simulink library "RxTxFixedPointLibrary"  (R2018a)
settings: Solver=VariableStepAuto  StartTime=0.0  StopTime=10.0  RelTol=1e-3
values from neighbouring files (symbols this model uses):
  AGCBarkerSymbols = 160 + 28    (= 188)    [modelSettings.m]
  coeff = rcosdesign(beta, span, sps, 'sqrt') * filterGain    [modelSettings.m]
  crcDecodeLag = length(crc32Poly) - 1 + 2    [modelSettings.m]
  CRCGeneratorLag = 34    [modelSettings.m]
  EQTrainingSymbols = 250    [modelSettings.m]
  K1 = fi(K1, 0)    [modelSettings.m]
  K2 = fi(K2, 0)    [modelSettings.m]
  numHeaderBits = 16    [modelSettings.m]
  numTrainingSamples = 250    [modelSettings.m]
  pLen = uint16(length(PreambleBarkersBits))    [modelSettings.m]
  RadioSampleRate = 1e6    (= 1000000)    [modelSettings.m]
  samplesPerSymbol = 4    [modelSettings.m]
  VibertiTracebackLength = 34 + 0    (= 34)    [modelSettings.m]
  xPreambleSeq = hPSKModTrain(seq)    [modelSettings.m]
undefined symbols (not defined in the file or in its folder): j
libraries: simulink x25, dsphdlfiltering x20, hdlsllib x10, commseqgen3 x4, commdigbbndpm3 x3, commcrc2 x2, commcnvcod2 x2, dspstat3 x1, commfilt2 x1, dspsigops x1
(part 2 of 3)

== system RxTxFixedPointLibrary/Receiver_HDL/Frame Recover/Barker Locate/Measure Phase Ambiguity ==
  data : Inport  OutDataTypeStr=int16
  trigger : Inport  Port=2
  validIn : Inport  Port=3
  Find Max and Set Output Shift : Subsystem
  HDL Opt Complex FIR4 : Subsystem  mask{Taps=xPreambleSeq(end:-1:1).'}
  HDL Opt Complex FIR5 : Subsystem  mask{Taps=exp(-j*pi/2).*xPreambleSeq(end:-1:1).'}
  HDL Opt Complex FIR6 : Subsystem  mask{Taps=exp(-j*pi).*xPreambleSeq(end:-1:1).'}
  HDL Opt Complex FIR7 : Subsystem  mask{Taps=exp(-j*pi*3/2).*xPreambleSeq(end:-1:1).'}
  Logical Operator : Logic  Inputs=5  AllPortsSameDT=off  OutDataTypeStr=boolean
  PA : Outport  InitialOutput=0
  wires:
  trigger/1 -> Logical Operator/5
  Logical Operator/1 -> Find Max and Set Output Shift/Enable
  HDL Opt Complex FIR7/2(validOut) -> Logical Operator/4
  HDL Opt Complex FIR6/2(validOut) -> Logical Operator/3
  HDL Opt Complex FIR5/2(validOut) -> Logical Operator/2
  HDL Opt Complex FIR4/2(validOut) -> Logical Operator/1
  validIn/1 -> HDL Opt Complex FIR6/2(validIn), HDL Opt Complex FIR7/2(validIn), HDL Opt Complex FIR5/2(validIn), HDL Opt Complex FIR4/2(validIn)
  Find Max and Set Output Shift/1(Out1) -> PA/1
  HDL Opt Complex FIR7/1(Out1) -> Find Max and Set Output Shift/4(In5)
  HDL Opt Complex FIR6/1(Out1) -> Find Max and Set Output Shift/3(In4)
  HDL Opt Complex FIR5/1(Out1) -> Find Max and Set Output Shift/2(In2)
  HDL Opt Complex FIR4/1(Out1) -> Find Max and Set Output Shift/1(In1)
  data/1 -> HDL Opt Complex FIR6/1(In1), HDL Opt Complex FIR7/1(In1), HDL Opt Complex FIR5/1(In1), HDL Opt Complex FIR4/1(In1)

== system RxTxFixedPointLibrary/Receiver_HDL/Frame Recover/Equalization and Demodulation/2 Bit Descrambler ==
  note: This is a special Descrambler which can process 2 bits at a time
  u1 : Inport
  reset : Inport  Port=2
  Demux1 : Demux  Outputs=2
  MATLAB Function : MATLAB Function  TreatAsAtomicUnit=on
  Mux : Mux  Inputs=2
  Selector1 : Selector  IndexOptions=Index vector (dialog)  Indices=find(polynom(2:end))  OutputSizes=1
  Selector2 : Selector  IndexOptions=Index vector (dialog)  Indices=find(polynom(2:end))  OutputSizes=1
  input_xor1 : Logic  Operator=XOR  IconShape=distinctive  AllPortsSameDT=off  OutDataTypeStr=boolean
  input_xor2 : Logic  Operator=XOR  IconShape=distinctive  AllPortsSameDT=off  OutDataTypeStr=boolean
  state_xor1 : Logic  Operator=XOR  Inputs=1  IconShape=distinctive  AllPortsSameDT=off  OutDataTypeStr=boolean
  state_xor2 : Logic  Operator=XOR  Inputs=1  IconShape=distinctive  AllPortsSameDT=off  OutDataTypeStr=boolean
  y1 : Outport  InitialOutput=0
  wires:
  Demux1/2 -> input_xor2/2  "data_in"
  Demux1/1 -> input_xor1/2
  Selector2/1 -> state_xor2/1
  Selector1/1 -> state_xor1/1
  input_xor1/1 -> Mux/1
  input_xor2/1 -> Mux/2
  state_xor2/1 -> input_xor2/1
  state_xor1/1 -> input_xor1/1
  Mux/1 -> y1/1
  MATLAB Function/2(bufferB) -> Selector2/1
  MATLAB Function/1(bufferA) -> Selector1/1
  reset/1 -> MATLAB Function/2(reset)
  u1/1 -> MATLAB Function/1(bits), Demux1/1

== system RxTxFixedPointLibrary/Receiver_HDL/Frame Recover/Equalization and Demodulation/DFE ==
  note: Generate training sequence when barker is found
  note: refTap=0 to disableEQ
  Trigger : Inport  PortDimensions=1
  data : Inport  Port=2  PortDimensions=1
      settings: SignalType=complex
  EQmu : Inport  Port=3
  DFE : Subsystem  mask{numFTaps=5, numBTaps=3, mu=0.01, refTap=2}
      mask prompts: numFTaps "Num Forward Taps"; numBTaps "Num Backward Taps"; mu "Step Size"; refTap "Reference Tap"
  Delay data so DFE can reset : Delay  DelayLength=1
  Delay ref so DFE can reset : Delay  DelayLength=1
  Equalizer : MATLAB Function  Commented=on  TreatAsAtomicUnit=on
  PN Sequence Generator : commseqgen3/PN Sequence Generator  poly='z^5 + z^3 + z^1 + 1'  ini_sta=[1 1 1 0 0]  outBitMaskSource=Dialog parameter  shift=0  outVarSiz=off  maxOutSizeMode=Dialog parameter  maxOutSize=[10 1]  Ts=-1  sampPerFrame=1  reset=on  bitPackedOutputs=on  outDataType=Smallest unsigned integer  numPackedBits=2  bitPackDataSigned=off  bitPackedOutDType=Smallest integer
      settings: SourceProductName=Communications System Toolbox
  Packeted To Unpacked : Subsystem
  QPSK Modulator Baseband : commdigbbndpm3/QPSK Modulator Baseband  InType=Bit  Enc=Binary  Ph=pi/4  outDtype=Fixed-point  outWordLen=16  outUDDataType=sfix(16)  outFracLenMode=User-defined  outFracLen=15  outDataTypeStr=fixdt(1,16,15)  outLastDataTypeStr=fixdt(1,16,15)
  Terminator1 : Terminator
  dataEQed : Outport
  start : Outport  Port=2
  wires:
  EQmu/1 -> DFE/4(EQmu)
  Delay ref so DFE can reset/1 -> DFE/3(training)
  Delay data so DFE can reset/1 -> DFE/2(dataIn)
  DFE/1(eqOut) -> dataEQed/1
  DFE/2(err) -> Terminator1/1
  Trigger/1 -> PN Sequence Generator/1, DFE/1(reset)
  DFE/3(start) -> start/1
  QPSK Modulator Baseband/1 -> Delay ref so DFE can reset/1
  Packeted To Unpacked/1(Out1) -> QPSK Modulator Baseband/1
  PN Sequence Generator/1 -> Packeted To Unpacked/1(In1)
  data/1 -> Delay data so DFE can reset/1

== system RxTxFixedPointLibrary/Receiver_HDL/Frame Recover/Frequency Recovery/Lock Detector ==
  ped : Inport
  Compare To Constant : simulink/Logic and Bit Operations/Compare To Constant  relop=<=  const=Threshold*WindowLength  OutDataTypeStr=boolean
  MATLAB Function : MATLAB Function  TreatAsAtomicUnit=on
  PED Error : Scope  Commented=on  NumInputPorts=3
  Pipeline Delay : Delay  DelayLength=1
  Sum of Elements : Sum  Inputs=+
  Tapped Delay : simulink/Discrete/Tapped Delay  vinit=0.0  samptime=-1  NumDelays=WindowLength  DelayOrder=Oldest  includeCurrent=off
  lock : Outport
  wires:
  ped/1 -> Pipeline Delay/1
  Tapped Delay/1 -> Sum of Elements/1
  Sum of Elements/1 -> PED Error/3, Compare To Constant/1
  Compare To Constant/1 -> lock/1, PED Error/2
  MATLAB Function/1(y) -> PED Error/1, Tapped Delay/1
  Pipeline Delay/1 -> MATLAB Function/1(u)

== system RxTxFixedPointLibrary/Receiver_HDL/Frame Recover/Frequency Recovery/Loop Filter ==
  note: Proportional-plus-Integrator Loop Filter,
      | Infinite DC Response to guarantee convergence
  note: This inflation is necessary
  e : Inport
  Add1 : Sum  RndMeth=Nearest  OutDataTypeStr=Inherit: Same as first input
  Add2 : Sum  OutDataTypeStr=Inherit: Same as first input
  Data Type Conversion : DataTypeConversion  OutDataTypeStr=fixdt(1,25,20)
  Delay : Delay  DelayLength=1
  Delay3 : Delay  DelayLength=1
  Delay4 : Delay  DelayLength=1
  K1 : Gain  Gain=K2  OutDataTypeStr=Inherit: Same as input
  K2 : Gain  Gain=K1  OutDataTypeStr=Inherit: Same as input
  Sum2 : Sum  OutDataTypeStr=Inherit: Same as first input
  v : Outport
  wires:
  Data Type Conversion/1 -> v/1
  Add2/1 -> Data Type Conversion/1, Delay4/1
  Delay4/1 -> Add2/2
  Delay3/1 -> Add2/1
  Sum2/1 -> Delay3/1
  Delay/1 -> Add1/1
  K2/1 -> Add1/2, Delay/1
  e/1 -> K1/1, K2/1
  Add1/1 -> Sum2/2
  K1/1 -> Sum2/1

== system RxTxFixedPointLibrary/Receiver_HDL/Frame Recover/Frequency Recovery/Loop Filter Configurable ==
  note: Proportional-plus-Integrator Loop Filter,
      | Infinite DC Response to guarantee convergence
  note: This inflation is necessary
  e : Inport
  LoopBW : Inport  Port=2
  Add1 : Sum  RndMeth=Nearest  OutDataTypeStr=Inherit: Same as first input
  Add2 : Sum  OutDataTypeStr=Inherit: Same as first input
  Data Type Conversion : DataTypeConversion  OutDataTypeStr=fixdt(1,25,20)
  Delay : Delay  DelayLength=1
  Delay3 : Delay  DelayLength=1
  Delay4 : Delay  DelayLength=1
  Direct Lookup Table (n-D) : LookupNDDirect  NumberOfTableDimensions=1  Table=K1  DiagnosticForOutOfRangeInput=Error
  Direct Lookup Table (n-D)1 : LookupNDDirect  NumberOfTableDimensions=1  Table=K2  DiagnosticForOutOfRangeInput=Error
  Product : Product  OutDataTypeStr=Inherit: Same as first input
  Product1 : Product  OutDataTypeStr=Inherit: Same as first input
  Sum2 : Sum  OutDataTypeStr=Inherit: Same as first input
  v : Outport
  wires:
  LoopBW/1 -> Direct Lookup Table (n-D)1/1, Direct Lookup Table (n-D)/1
  Direct Lookup Table (n-D)1/1 -> Product1/2
  Direct Lookup Table (n-D)/1 -> Product/2
  Data Type Conversion/1 -> v/1
  Add2/1 -> Data Type Conversion/1, Delay4/1
  Delay4/1 -> Add2/2
  Delay3/1 -> Add2/1
  Sum2/1 -> Delay3/1
  Delay/1 -> Add1/1
  Product1/1 -> Add1/2, Delay/1
  e/1 -> Product/1, Product1/1
  Add1/1 -> Sum2/2
  Product/1 -> Sum2/1

== system RxTxFixedPointLibrary/Receiver_HDL/Frame Recover/Frequency Recovery/Phase Shift FP ==
  note: Sign Comes from original
      | loop filter design
  In1 : Inport
  Phi : Inport  Port=2
  Cosine HDL Optimized : hdlsllib/Lookup Tables/Cosine HDL Optimized  OutputFormula=exp(j*2*pi*u)  NumDataPoints=256  TableDataTypeStr=fixdt(0,31,20)  SimulateLUTROMDelay=off
      settings: SourceProductName=HDL Coder  SourceProductBaseCode=HD
  Gain : Gain  Gain=-1/(2*pi)  ParamDataTypeStr=fixdt(1,25,20)  OutDataTypeStr=fixdt(1,16,12)  SaturateOnIntegerOverflow=on
  Product : Product  OutDataTypeStr=fixdt(1,16,13)  SaturateOnIntegerOverflow=on
  Out1 : Outport
  wires:
  Gain/1 -> Cosine HDL Optimized/1
  Phi/1 -> Gain/1
  In1/1 -> Product/1
  Cosine HDL Optimized/1 -> Product/2
  Product/1 -> Out1/1

== system RxTxFixedPointLibrary/Receiver_HDL/Frame Recover/Gardner Timing Recovery/Gardner TED Blocks ==
  note: This is for QPSK and 4 SamplesPerSymbol ONLY
  note: An input of 4 should not
      | happen unless the input is all zeros
  data : Inport
  strobe : Inport  Port=2
  Add : Sum  OutDataTypeStr=fixdt(1,16,15)
  Check Only Strobe Condition : simulink/Logic and Bit Operations/Compare To Constant  relop===  const=uint8(1)  OutDataTypeStr=boolean
  Complex to Real-Imag : ComplexToRealImag
  Constant : Constant  Value=0  OutDataTypeStr=Inherit: Inherit via back propagation  SampleTime=-1
  Display : Display
  Imag Error : Subsystem
  Logical Operator : Logic  AllPortsSameDT=off  OutDataTypeStr=boolean
  Map [0,1,2,3,4] to [0,1,2,2,2] : LookupNDDirect  NumberOfTableDimensions=1  Table=[0 1 2 2 2]  DiagnosticForOutOfRangeInput=Error  TableDataTypeStr=uint8
  Real Error : Subsystem
  Strobe Buffer1 : simulink/Discrete/Tapped Delay  vinit=0.0  samptime=-1  NumDelays=samplesPerSymbol-1  DelayOrder=Oldest  includeCurrent=on
  Sum of Elements1 : Sum  Inputs=+  OutDataTypeStr=int8
  Switch : Switch  Criteria=u2 ~= 0  SaturateOnIntegerOverflow=on
  e : Outport
  wires:
  Logical Operator/1 -> Switch/2
  Add/1 -> Switch/1
  Imag Error/1(Out1) -> Add/2
  Real Error/1(Out1) -> Add/1
  Strobe Buffer1/1 -> Sum of Elements1/1
  Map [0,1,2,3,4] to [0,1,2,2,2]/1 -> Real Error/2(strobe sum), Imag Error/2(strobe sum)
  data/1 -> Complex to Real-Imag/1
  Complex to Real-Imag/1 -> Real Error/1(data)
  Constant/1 -> Switch/3
  Check Only Strobe Condition/1 -> Logical Operator/1
  Sum of Elements1/1 -> Map [0,1,2,3,4] to [0,1,2,2,2]/1, Check Only Strobe Condition/1, Display/1
  Complex to Real-Imag/2 -> Imag Error/1(data)
  strobe/1 -> Logical Operator/2, Strobe Buffer1/1
  Switch/1 -> e/1

== system RxTxFixedPointLibrary/Receiver_HDL/Frame Recover/Gardner Timing Recovery/InterpControl_Blocks1 ==
  note: Mu is always positive
  note: e<<1/SPS
  e : Inport
  1/SPS1 : Constant  Value=fi(1/samplesPerSymbol,0,2,2)  OutDataTypeStr=fixdt(0,2,2)  SampleTime=-1
  Add1 : Sum  OutDataTypeStr=fixdt(0,16,16)
  Calculate New mu : Subsystem
  Display{,1..3} (4 alike) : Display
  Mod 1 : Subsystem
  NCOCounter State : Delay  DelayLength=1  InitialCondition=0
  Subtract1 : Sum  Inputs=-+  OutDataTypeStr=Inherit: Same as first input
  Update mu on strobe : Switch  Criteria=u2 > Threshold
  saved mu : Delay  DelayLength=1
  strobe == W>NCOCounter : RelationalOperator  Operator=>  OutDataTypeStr=boolean  RndMeth=Nearest
  strobe : Outport
  mu : Outport  Port=2
  wires:
  Add1/1 -> Subtract1/1, Display2/1, strobe == W>NCOCounter/1, Calculate New mu/1(W)
  1/SPS1/1 -> Add1/2
  Mod 1/1(Out1) -> NCOCounter State/1
  Subtract1/1 -> Mod 1/1(In1)
  NCOCounter State/1 -> Calculate New mu/2(NCOCounter), strobe == W>NCOCounter/2, Display1/1, Subtract1/2
  e/1 -> Add1/1
  Calculate New mu/1(mu) -> Update mu on strobe/1, Display/1
  saved mu/1 -> Update mu on strobe/3
  Update mu on strobe/1 -> saved mu/1, mu/1, Display3/1
  strobe == W>NCOCounter/1 -> strobe/1, Update mu on strobe/2

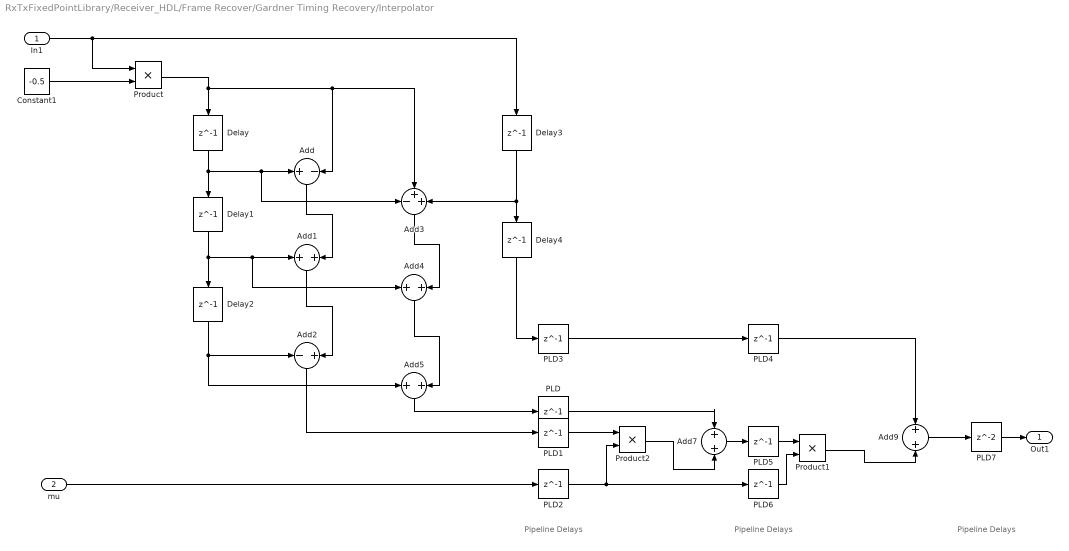
== system RxTxFixedPointLibrary/Receiver_HDL/Frame Recover/Gardner Timing Recovery/Interpolator ==
  note: Pipeline Delays
  note: Pipeline Delays
  note: Pipeline Delays
  In1 : Inport
  mu : Inport  Port=2
  Add : Sum  Inputs=+-  OutDataTypeStr=Inherit: Same as first input
  Add{1,4..5,7} (4 alike) : Sum
  Add2 : Sum  Inputs=-+
  Add3 : Sum  Inputs=-++
  Add9 : Sum  OutDataTypeStr=fixdt(1,16,10)
  Constant1 : Constant  Value=-0.5  OutDataTypeStr=fixdt(1,2,2)  SampleTime=-1
  Delay{,1..4} (5 alike) : Delay  DelayLength=1
  PLD{,1..6} (7 alike) : Delay  DelayLength=1
  PLD7 : Delay
  Product : Product  OutDataTypeStr=fixdt(1,16,14)
  Product1 : Product
  Product2 : Product  OutDataTypeStr=fixdt(1,16,10)
  Out1 : Outport
  wires:
  PLD7/1 -> Out1/1
  PLD6/1 -> Product1/2
  PLD5/1 -> Product1/1
  PLD4/1 -> Add9/1
  PLD3/1 -> PLD4/1
  PLD2/1 -> PLD6/1, Product2/2
  PLD1/1 -> Product2/1
  PLD/1 -> Add7/1
  Constant1/1 -> Product/2
  Product1/1 -> Add9/2
  Add7/1 -> PLD5/1
  Delay4/1 -> PLD3/1
  Delay3/1 -> Add3/3, Delay4/1
  Add9/1 -> PLD7/1
  Product2/1 -> Add7/2
  Add5/1 -> PLD/1
  mu/1 -> PLD2/1
  Add2/1 -> PLD1/1
  Add4/1 -> Add5/2
  Add3/1 -> Add4/2
  Add1/1 -> Add2/2
  Delay2/1 -> Add2/1, Add5/1
  Add/1 -> Add1/2
  Delay1/1 -> Delay2/1, Add1/1, Add4/1
  Delay/1 -> Delay1/1, Add/1, Add3/1
  Product/1 -> Delay/1, Add/2, Add3/2
  In1/1 -> Product/1, Delay3/1

== system RxTxFixedPointLibrary/Receiver_HDL/Frame Recover/Gardner Timing Recovery/LoopFilter1 ==
  e : Inport
  Delay1 : Delay  DelayLength=1
  Delay2 : Delay  DelayLength=1
  Proportional Gain : Gain  Gain=fi(ProportionalGain,1,16,15)  OutDataTypeStr=fixdt(1,16,24)
  v : Outport
  wires:
  Delay1/1 -> v/1
  Delay2/1 -> Proportional Gain/1
  Proportional Gain/1 -> Delay1/1
  e/1 -> Delay2/1

== system RxTxFixedPointLibrary/Receiver_HDL/Frame Recover/Gardner Timing Recovery/TED Lock Detector ==
  ted : Inport
  Compare To Constant : simulink/Logic and Bit Operations/Compare To Constant  relop=<=  const=Threshold*WindowLength  OutDataTypeStr=boolean
  MATLAB Function : MATLAB Function  TreatAsAtomicUnit=on
  Pipeline Delay : Delay  DelayLength=1
  Sum of Elements : Sum  Inputs=+
  TED Error : Scope  Commented=on  NumInputPorts=3
  Tapped Delay : simulink/Discrete/Tapped Delay  vinit=0.0  samptime=-1  NumDelays=WindowLength  DelayOrder=Oldest  includeCurrent=off
  lock : Outport
  wires:
  ted/1 -> Pipeline Delay/1
  Tapped Delay/1 -> Sum of Elements/1
  Sum of Elements/1 -> TED Error/3, Compare To Constant/1
  Compare To Constant/1 -> lock/1, TED Error/2
  MATLAB Function/1(y) -> TED Error/1, Tapped Delay/1
  Pipeline Delay/1 -> MATLAB Function/1(u)

== system RxTxFixedPointLibrary/Receiver_HDL/Frame Recover/Manage Error Signals/Subsystem ==
  <status> : Inport
  <s1> : Inport  Port=2
  <s2> : Inport  Port=3
  Enable : EnablePort
  DEBUG: Header : MATLAB Function  Commented=on  TreatAsAtomicUnit=on
  wires:
  <s1>/1 -> DEBUG: Header/2(h1)
  <status>/1 -> DEBUG: Header/1(status)
  <s2>/1 -> DEBUG: Header/3(h2)

== system RxTxFixedPointLibrary/Receiver_HDL/Viterbi Decode/Buffer/DEBUG: Vitberi Check ==
  In1 : Inport
  In2 : Inport  Port=2
  In3 : Inport  Port=3
  In4 : Inport  Port=4
  Allow Viterbi Reset2 : Delay  DelayLength=1
  Allow Viterbi Reset3 : Delay  DelayLength=34
  Allow Viterbi Reset4 : Delay  DelayLength=1
  MATLAB Function2 : MATLAB Function  TreatAsAtomicUnit=on
  wires:
  In3/1 -> Allow Viterbi Reset2/1
  In1/1 -> MATLAB Function2/1(bits)
  In2/1 -> Allow Viterbi Reset4/1
  Allow Viterbi Reset2/1 -> MATLAB Function2/3(reset)
  In4/1 -> Allow Viterbi Reset3/1
  Allow Viterbi Reset3/1 -> MATLAB Function2/4(crc)
  Allow Viterbi Reset4/1 -> MATLAB Function2/2(enable)

== system RxTxFixedPointLibrary/Transmitter_HDL/Packet Generation/Payload/Enable Latch ==
  note: This block will latch when start flag is high and then latch low when end flag arrives
  mode : Inport
  start : Inport  Port=2
  end : Inport  Port=3
  Compare To Constant : simulink/Logic and Bit Operations/Compare To Constant  relop=>=  const=uint8(1)  OutDataTypeStr=boolean
  Compare To Constant1 : simulink/Logic and Bit Operations/Compare To Constant  relop===  const=uint8(1)  OutDataTypeStr=boolean
  HDL Counter1 : hdlsllib/Sources/HDL Counter  CountType=Count limited  CountInit=0  CountStep=1  CountMax=1  CountFromType=Initial value  CountFrom=0  CountResetPort=on  CountLoadPort=off  CountEnbPort=on  CountDirPort=off  CountDataType=Unsigned  CountWordLen=8  CountFracLen=0  CountSampTime=1
      settings: SourceProductBaseCode=HD
  Logical Operator : Logic  AllPortsSameDT=off  OutDataTypeStr=boolean
  Logical Operator1 : Logic  AllPortsSameDT=off  OutDataTypeStr=boolean
  Logical Operator2 : Logic  Operator=OR  AllPortsSameDT=off  OutDataTypeStr=boolean
  MATLAB Function : MATLAB Function  Commented=on  TreatAsAtomicUnit=on
  Terminator : Terminator  Commented=on
  valid : Outport
  wires:
  mode/1 -> Compare To Constant/1
  Compare To Constant/1 -> Logical Operator1/1, Logical Operator/1
  start/1 -> MATLAB Function/1(startpacket), Logical Operator/2
  end/1 -> MATLAB Function/2(endpacket), Logical Operator1/2
  HDL Counter1/1 -> Compare To Constant1/1
  Logical Operator1/1 -> HDL Counter1/1
  Logical Operator/1 -> Logical Operator2/1, HDL Counter1/2
  Compare To Constant1/1 -> Logical Operator2/2
  MATLAB Function/1(outEnable) -> Terminator/1
  Logical Operator2/1 -> valid/1

== system RxTxFixedPointLibrary/Transmitter_HDL/Packet Generation/Payload/HDL Scrambler 2 bits ==
  bitsIn : Inport
  reset : Inport  Port=2
  Buffer Manage : MATLAB Function  TreatAsAtomicUnit=on
  Delay : Delay  DelayLength=1  InitialCondition=false
  Delay1 : Delay  DelayLength=1  InitialCondition=false
  Demux : Demux  Outputs=2
  Display1 : Display
  Display3 : Display
  Mux : Mux  Inputs=2
  Mux1 : Mux  Inputs=2
  Selector : Selector  IndexOptions=Index vector (dialog)  Indices=find(poly(2:end))  OutputSizes=1
  Selector1 : Selector  IndexOptions=Index vector (dialog)  Indices=1+find(poly(2:end))  OutputSizes=1
  state_xor1 : Logic  Operator=XOR  IconShape=distinctive  AllPortsSameDT=off  OutDataTypeStr=boolean
  state_xor2 : Logic  Operator=XOR  Inputs=1  IconShape=distinctive  AllPortsSameDT=off  OutDataTypeStr=boolean
  state_xor3 : Logic  Operator=XOR  Inputs=1  IconShape=distinctive  AllPortsSameDT=off  OutDataTypeStr=boolean
  state_xor4 : Logic  Operator=XOR  IconShape=distinctive  AllPortsSameDT=off  OutDataTypeStr=boolean
  bitsOut : Outport
  wires:
  bitsIn/1 -> Display1/1, Demux/1
  Selector/1 -> state_xor2/1
  state_xor2/1 -> Display3/1, state_xor1/1
  Demux/1 -> state_xor1/2
  state_xor1/1 -> Mux1/2, Mux/1, Delay/1
  Mux/1 -> bitsOut/1
  Mux1/1 -> Selector1/1
  Buffer Manage/1(outBuffer) -> Mux1/1, Selector/1
  Selector1/1 -> state_xor3/1
  state_xor3/1 -> state_xor4/1
  Demux/2 -> state_xor4/2
  state_xor4/1 -> Delay1/1, Mux/2
  Delay/1 -> Buffer Manage/1(bit1)
  reset/1 -> Buffer Manage/3(reset)
  Delay1/1 -> Buffer Manage/2(bit2)

== system RxTxFixedPointLibrary/Transmitter_HDL/Packet Generation/Payload/Subsystem ==
  In1 : Inport
  In2 : Inport  Port=2
  Logical Operator : Logic  Operator=OR  Inputs=3  AllPortsSameDT=off  OutDataTypeStr=boolean
  MATLAB Function3 : MATLAB Function  TreatAsAtomicUnit=on
  Out1 : Outport
  wires:
  In2/1 -> Logical Operator/3, MATLAB Function3/2(done)
  In1/1 -> Logical Operator/1, MATLAB Function3/1(start)
  MATLAB Function3/1(enable) -> Logical Operator/2
  Logical Operator/1 -> Out1/1

== system RxTxFixedPointLibrary/Transmitter_HDL/Packet Generation/Preamble/Unpack1 ==
  In1 : Inport
  Data Type Conversion : DataTypeConversion  OutDataTypeStr=boolean
  Extract Bits : simulink/Logic and Bit Operations/Extract Bits  bitsToExtract=Range of bits  numBits=8  bitIdxRange=[1]  outScalingMode=Treat bit field as an integer
      settings: SourceProductName=Simulink
  Extract Bits1 : simulink/Logic and Bit Operations/Extract Bits  bitsToExtract=Range of bits  numBits=8  bitIdxRange=[0]  outScalingMode=Treat bit field as an integer
      settings: SourceProductName=Simulink
  Vector Concatenate : Concatenate
  Out1 : Outport
  wires:
  In1/1 -> Extract Bits1/1, Extract Bits/1
  Extract Bits/1 -> Vector Concatenate/1
  Extract Bits1/1 -> Vector Concatenate/2
  Vector Concatenate/1 -> Data Type Conversion/1
  Data Type Conversion/1 -> Out1/1

== system RxTxFixedPointLibrary/Transmitter_HDL/Packet Generation/Random Data/Unpack ==
  In1 : Inport
  Data Type Conversion : DataTypeConversion  OutDataTypeStr=boolean
  Extract Bits : simulink/Logic and Bit Operations/Extract Bits  bitsToExtract=Range of bits  numBits=8  bitIdxRange=[0]  outScalingMode=Treat bit field as an integer
      settings: SourceProductName=Simulink
  Extract Bits1 : simulink/Logic and Bit Operations/Extract Bits  bitsToExtract=Range of bits  numBits=8  bitIdxRange=[1]  outScalingMode=Treat bit field as an integer
      settings: SourceProductName=Simulink
  Vector Concatenate : Concatenate
  Out1 : Outport
  wires:
  In1/1 -> Extract Bits1/1, Extract Bits/1
  Extract Bits/1 -> Vector Concatenate/1
  Extract Bits1/1 -> Vector Concatenate/2
  Vector Concatenate/1 -> Data Type Conversion/1
  Data Type Conversion/1 -> Out1/1

== system RxTxFixedPointLibrary/Receiver_HDL/Frame Recover/Barker Locate/Measure Phase Ambiguity/Find Max and Set Output Shift ==
  In1 : Inport
  In2 : Inport  Port=2
  In4 : Inport  Port=3
  In5 : Inport  Port=4
  Enable : EnablePort
  Complex to Real-Imag{,1..3} (4 alike) : ComplexToRealImag  Output=Imag
  Direct Lookup Table (n-D) : LookupNDDirect  NumberOfTableDimensions=1  Table=exp(-(0:pi/2:(pi*3/2)) .* 1i).'  DiagnosticForOutOfRangeInput=Error  TableDataTypeStr=fixdt(1,16,13)
  Display : Display
  Display1 : Display
  Maximum : dspstat3/Maximum  operation=maximum  fcn=Index  indexBase=Zero  operateOver=Each column  Dimension=1  InputProcessing=Columns as channels (frame based)  reset=None  roiEnable=off  roiType=Rectangles  roiPortion=Entire ROI  roiOutput=Individual statistics for each ROI  roiFlag=off  roundingMode=Floor  overflowMode=off  accumDataTypeStr=Inherit: Same as product output  accumLastDataTypeStr=Inherit: Same as product output
  Vector Concatenate : Concatenate  NumInputs=4
  Vector Concatenate1 : Concatenate  NumInputs=4
  Out1 : Outport  InitialOutput=0
  wires:
  Complex to Real-Imag/1 -> Vector Concatenate/1
  Complex to Real-Imag2/1 -> Vector Concatenate/3
  Complex to Real-Imag3/1 -> Vector Concatenate/4
  Complex to Real-Imag1/1 -> Vector Concatenate/2
  Vector Concatenate1/1 -> Display/1
  Vector Concatenate/1 -> Display1/1, Maximum/1
  Maximum/1 -> Direct Lookup Table (n-D)/1
  In1/1 -> Complex to Real-Imag/1, Vector Concatenate1/1
  In5/1 -> Complex to Real-Imag3/1, Vector Concatenate1/4
  In2/1 -> Complex to Real-Imag1/1, Vector Concatenate1/2
  In4/1 -> Complex to Real-Imag2/1, Vector Concatenate1/3
  Direct Lookup Table (n-D)/1 -> Out1/1

== system RxTxFixedPointLibrary/Receiver_HDL/Frame Recover/Barker Locate/Measure Phase Ambiguity/HDL Opt Complex FIR4 ==
  In1 : Inport
  validIn : Inport  Port=2
  Add : Sum  Inputs=+-  AccumDataTypeStr=fixdt(1,16,0)
  Complex to Real-Imag : ComplexToRealImag
  Discrete FIR Filter HDL Optimized : dsphdlfiltering/Discrete FIR Filter HDL Optimized  Numerator=real(Taps)  Sharing=off  SharingFactor=2  SimulateUsing=Code generation  roundingMode=Floor  overflowMode=off  CoefficientsDataTypeStr=Inherit: Same word length as input  CoefficientsMin=[]  CoefficientsMax=[]  OutputDataTypeStr=fixdt(1,16,0)  OutputMin=[]  OutputMax=[]  ValidInPort=on  ReadyPort=off
      settings: SourceProductName=DSP System Toolbox  SourceProductBaseCode=DS
  Discrete FIR Filter HDL Optimized1 : dsphdlfiltering/Discrete FIR Filter HDL Optimized  Numerator=imag(Taps)  Sharing=off  SharingFactor=2  SimulateUsing=Code generation  roundingMode=Floor  overflowMode=off  CoefficientsDataTypeStr=Inherit: Same word length as input  CoefficientsMin=[]  CoefficientsMax=[]  OutputDataTypeStr=fixdt(1,16,0)  OutputMin=[]  OutputMax=[]  ValidInPort=on  ReadyPort=off
      settings: SourceProductName=DSP System Toolbox  SourceProductBaseCode=DS
  Discrete FIR Filter HDL Optimized2 : dsphdlfiltering/Discrete FIR Filter HDL Optimized  Numerator=real(Taps)  Sharing=off  SharingFactor=2  SimulateUsing=Code generation  roundingMode=Floor  overflowMode=off  CoefficientsDataTypeStr=Inherit: Same word length as input  CoefficientsMin=[]  CoefficientsMax=[]  OutputDataTypeStr=fixdt(1,16,0)  OutputMin=[]  OutputMax=[]  ValidInPort=on  ReadyPort=off
      settings: SourceProductName=DSP System Toolbox  SourceProductBaseCode=DS
  Discrete FIR Filter HDL Optimized3 : dsphdlfiltering/Discrete FIR Filter HDL Optimized  Numerator=imag(Taps)  Sharing=off  SharingFactor=2  SimulateUsing=Code generation  roundingMode=Floor  overflowMode=off  CoefficientsDataTypeStr=Inherit: Same word length as input  CoefficientsMin=[]  CoefficientsMax=[]  OutputDataTypeStr=fixdt(1,16,0)  OutputMin=[]  OutputMax=[]  ValidInPort=on  ReadyPort=off
      settings: SourceProductName=DSP System Toolbox  SourceProductBaseCode=DS
  Logical Operator : Logic  Inputs=4  AllPortsSameDT=off  OutDataTypeStr=boolean
  Real-Imag to Complex : RealImagToComplex
  Subtract : Sum  OutDataTypeStr=int16
  Out1 : Outport
  validOut : Outport  Port=2
  wires:
  Add/1 -> Real-Imag to Complex/1
  Subtract/1 -> Real-Imag to Complex/2
  Real-Imag to Complex/1 -> Out1/1
  Discrete FIR Filter HDL Optimized3/1 -> Subtract/2
  Discrete FIR Filter HDL Optimized2/1 -> Subtract/1
  Complex to Real-Imag/2 -> Discrete FIR Filter HDL Optimized1/1, Discrete FIR Filter HDL Optimized2/1
  Discrete FIR Filter HDL Optimized3/2 -> Logical Operator/4
  Discrete FIR Filter HDL Optimized2/2 -> Logical Operator/3
  Complex to Real-Imag/1 -> Discrete FIR Filter HDL Optimized/1, Discrete FIR Filter HDL Optimized3/1
  In1/1 -> Complex to Real-Imag/1
  validIn/1 -> Discrete FIR Filter HDL Optimized/2, Discrete FIR Filter HDL Optimized1/2, Discrete FIR Filter HDL Optimized2/2, Discrete FIR Filter HDL Optimized3/2
  Discrete FIR Filter HDL Optimized1/1 -> Add/2
  Discrete FIR Filter HDL Optimized1/2 -> Logical Operator/2
  Discrete FIR Filter HDL Optimized/2 -> Logical Operator/1
  Logical Operator/1 -> validOut/1
  Discrete FIR Filter HDL Optimized/1 -> Add/1

== system RxTxFixedPointLibrary/Receiver_HDL/Frame Recover/Barker Locate/Measure Phase Ambiguity/HDL Opt Complex FIR5 ==
  In1 : Inport
  validIn : Inport  Port=2
  Add : Sum  Inputs=+-  AccumDataTypeStr=fixdt(1,16,0)
  Complex to Real-Imag : ComplexToRealImag
  Discrete FIR Filter HDL Optimized : dsphdlfiltering/Discrete FIR Filter HDL Optimized  Numerator=real(Taps)  Sharing=off  SharingFactor=2  SimulateUsing=Code generation  roundingMode=Floor  overflowMode=off  CoefficientsDataTypeStr=Inherit: Same word length as input  CoefficientsMin=[]  CoefficientsMax=[]  OutputDataTypeStr=fixdt(1,16,0)  OutputMin=[]  OutputMax=[]  ValidInPort=on  ReadyPort=off
      settings: SourceProductName=DSP System Toolbox  SourceProductBaseCode=DS
  Discrete FIR Filter HDL Optimized1 : dsphdlfiltering/Discrete FIR Filter HDL Optimized  Numerator=imag(Taps)  Sharing=off  SharingFactor=2  SimulateUsing=Code generation  roundingMode=Floor  overflowMode=off  CoefficientsDataTypeStr=Inherit: Same word length as input  CoefficientsMin=[]  CoefficientsMax=[]  OutputDataTypeStr=fixdt(1,16,0)  OutputMin=[]  OutputMax=[]  ValidInPort=on  ReadyPort=off
      settings: SourceProductName=DSP System Toolbox  SourceProductBaseCode=DS
  Discrete FIR Filter HDL Optimized2 : dsphdlfiltering/Discrete FIR Filter HDL Optimized  Numerator=real(Taps)  Sharing=off  SharingFactor=2  SimulateUsing=Code generation  roundingMode=Floor  overflowMode=off  CoefficientsDataTypeStr=Inherit: Same word length as input  CoefficientsMin=[]  CoefficientsMax=[]  OutputDataTypeStr=fixdt(1,16,0)  OutputMin=[]  OutputMax=[]  ValidInPort=on  ReadyPort=off
      settings: SourceProductName=DSP System Toolbox  SourceProductBaseCode=DS
  Discrete FIR Filter HDL Optimized3 : dsphdlfiltering/Discrete FIR Filter HDL Optimized  Numerator=imag(Taps)  Sharing=off  SharingFactor=2  SimulateUsing=Code generation  roundingMode=Floor  overflowMode=off  CoefficientsDataTypeStr=Inherit: Same word length as input  CoefficientsMin=[]  CoefficientsMax=[]  OutputDataTypeStr=fixdt(1,16,0)  OutputMin=[]  OutputMax=[]  ValidInPort=on  ReadyPort=off
      settings: SourceProductName=DSP System Toolbox  SourceProductBaseCode=DS
  Logical Operator : Logic  Inputs=4  AllPortsSameDT=off  OutDataTypeStr=boolean
  Real-Imag to Complex : RealImagToComplex
  Subtract : Sum  OutDataTypeStr=int16
  Out1 : Outport
  validOut : Outport  Port=2
  wires:
  Add/1 -> Real-Imag to Complex/1
  Subtract/1 -> Real-Imag to Complex/2
  Real-Imag to Complex/1 -> Out1/1
  Discrete FIR Filter HDL Optimized3/1 -> Subtract/2
  Discrete FIR Filter HDL Optimized2/1 -> Subtract/1
  Complex to Real-Imag/2 -> Discrete FIR Filter HDL Optimized1/1, Discrete FIR Filter HDL Optimized2/1
  Discrete FIR Filter HDL Optimized3/2 -> Logical Operator/4
  Discrete FIR Filter HDL Optimized2/2 -> Logical Operator/3
  Complex to Real-Imag/1 -> Discrete FIR Filter HDL Optimized/1, Discrete FIR Filter HDL Optimized3/1
  In1/1 -> Complex to Real-Imag/1
  validIn/1 -> Discrete FIR Filter HDL Optimized/2, Discrete FIR Filter HDL Optimized1/2, Discrete FIR Filter HDL Optimized2/2, Discrete FIR Filter HDL Optimized3/2
  Discrete FIR Filter HDL Optimized1/1 -> Add/2
  Discrete FIR Filter HDL Optimized1/2 -> Logical Operator/2
  Discrete FIR Filter HDL Optimized/2 -> Logical Operator/1
  Logical Operator/1 -> validOut/1
  Discrete FIR Filter HDL Optimized/1 -> Add/1

== system RxTxFixedPointLibrary/Receiver_HDL/Frame Recover/Barker Locate/Measure Phase Ambiguity/HDL Opt Complex FIR6 ==
  In1 : Inport
  validIn : Inport  Port=2
  Add : Sum  Inputs=+-  AccumDataTypeStr=fixdt(1,16,0)
  Complex to Real-Imag : ComplexToRealImag
  Discrete FIR Filter HDL Optimized : dsphdlfiltering/Discrete FIR Filter HDL Optimized  Numerator=real(Taps)  Sharing=off  SharingFactor=2  SimulateUsing=Code generation  roundingMode=Floor  overflowMode=off  CoefficientsDataTypeStr=Inherit: Same word length as input  CoefficientsMin=[]  CoefficientsMax=[]  OutputDataTypeStr=fixdt(1,16,0)  OutputMin=[]  OutputMax=[]  ValidInPort=on  ReadyPort=off
      settings: SourceProductName=DSP System Toolbox  SourceProductBaseCode=DS
  Discrete FIR Filter HDL Optimized1 : dsphdlfiltering/Discrete FIR Filter HDL Optimized  Numerator=imag(Taps)  Sharing=off  SharingFactor=2  SimulateUsing=Code generation  roundingMode=Floor  overflowMode=off  CoefficientsDataTypeStr=Inherit: Same word length as input  CoefficientsMin=[]  CoefficientsMax=[]  OutputDataTypeStr=fixdt(1,16,0)  OutputMin=[]  OutputMax=[]  ValidInPort=on  ReadyPort=off
      settings: SourceProductName=DSP System Toolbox  SourceProductBaseCode=DS
  Discrete FIR Filter HDL Optimized2 : dsphdlfiltering/Discrete FIR Filter HDL Optimized  Numerator=real(Taps)  Sharing=off  SharingFactor=2  SimulateUsing=Code generation  roundingMode=Floor  overflowMode=off  CoefficientsDataTypeStr=Inherit: Same word length as input  CoefficientsMin=[]  CoefficientsMax=[]  OutputDataTypeStr=fixdt(1,16,0)  OutputMin=[]  OutputMax=[]  ValidInPort=on  ReadyPort=off
      settings: SourceProductName=DSP System Toolbox  SourceProductBaseCode=DS
  Discrete FIR Filter HDL Optimized3 : dsphdlfiltering/Discrete FIR Filter HDL Optimized  Numerator=imag(Taps)  Sharing=off  SharingFactor=2  SimulateUsing=Code generation  roundingMode=Floor  overflowMode=off  CoefficientsDataTypeStr=Inherit: Same word length as input  CoefficientsMin=[]  CoefficientsMax=[]  OutputDataTypeStr=fixdt(1,16,0)  OutputMin=[]  OutputMax=[]  ValidInPort=on  ReadyPort=off
      settings: SourceProductName=DSP System Toolbox  SourceProductBaseCode=DS
  Logical Operator : Logic  Inputs=4  AllPortsSameDT=off  OutDataTypeStr=boolean
  Real-Imag to Complex : RealImagToComplex
  Subtract : Sum  OutDataTypeStr=int16
  Out1 : Outport
  validOut : Outport  Port=2
  wires:
  Add/1 -> Real-Imag to Complex/1
  Subtract/1 -> Real-Imag to Complex/2
  Real-Imag to Complex/1 -> Out1/1
  Discrete FIR Filter HDL Optimized3/1 -> Subtract/2
  Discrete FIR Filter HDL Optimized2/1 -> Subtract/1
  Complex to Real-Imag/2 -> Discrete FIR Filter HDL Optimized1/1, Discrete FIR Filter HDL Optimized2/1
  Discrete FIR Filter HDL Optimized3/2 -> Logical Operator/4
  Discrete FIR Filter HDL Optimized2/2 -> Logical Operator/3
  Complex to Real-Imag/1 -> Discrete FIR Filter HDL Optimized/1, Discrete FIR Filter HDL Optimized3/1
  In1/1 -> Complex to Real-Imag/1
  validIn/1 -> Discrete FIR Filter HDL Optimized/2, Discrete FIR Filter HDL Optimized1/2, Discrete FIR Filter HDL Optimized2/2, Discrete FIR Filter HDL Optimized3/2
  Discrete FIR Filter HDL Optimized1/1 -> Add/2
  Discrete FIR Filter HDL Optimized1/2 -> Logical Operator/2
  Discrete FIR Filter HDL Optimized/2 -> Logical Operator/1
  Logical Operator/1 -> validOut/1
  Discrete FIR Filter HDL Optimized/1 -> Add/1

== system RxTxFixedPointLibrary/Receiver_HDL/Frame Recover/Barker Locate/Measure Phase Ambiguity/HDL Opt Complex FIR7 ==
  In1 : Inport
  validIn : Inport  Port=2
  Add : Sum  Inputs=+-  AccumDataTypeStr=fixdt(1,16,0)
  Complex to Real-Imag : ComplexToRealImag
  Discrete FIR Filter HDL Optimized : dsphdlfiltering/Discrete FIR Filter HDL Optimized  Numerator=real(Taps)  Sharing=off  SharingFactor=2  SimulateUsing=Code generation  roundingMode=Floor  overflowMode=off  CoefficientsDataTypeStr=Inherit: Same word length as input  CoefficientsMin=[]  CoefficientsMax=[]  OutputDataTypeStr=fixdt(1,16,0)  OutputMin=[]  OutputMax=[]  ValidInPort=on  ReadyPort=off
      settings: SourceProductName=DSP System Toolbox  SourceProductBaseCode=DS
  Discrete FIR Filter HDL Optimized1 : dsphdlfiltering/Discrete FIR Filter HDL Optimized  Numerator=imag(Taps)  Sharing=off  SharingFactor=2  SimulateUsing=Code generation  roundingMode=Floor  overflowMode=off  CoefficientsDataTypeStr=Inherit: Same word length as input  CoefficientsMin=[]  CoefficientsMax=[]  OutputDataTypeStr=fixdt(1,16,0)  OutputMin=[]  OutputMax=[]  ValidInPort=on  ReadyPort=off
      settings: SourceProductName=DSP System Toolbox  SourceProductBaseCode=DS
  Discrete FIR Filter HDL Optimized2 : dsphdlfiltering/Discrete FIR Filter HDL Optimized  Numerator=real(Taps)  Sharing=off  SharingFactor=2  SimulateUsing=Code generation  roundingMode=Floor  overflowMode=off  CoefficientsDataTypeStr=Inherit: Same word length as input  CoefficientsMin=[]  CoefficientsMax=[]  OutputDataTypeStr=fixdt(1,16,0)  OutputMin=[]  OutputMax=[]  ValidInPort=on  ReadyPort=off
      settings: SourceProductName=DSP System Toolbox  SourceProductBaseCode=DS
  Discrete FIR Filter HDL Optimized3 : dsphdlfiltering/Discrete FIR Filter HDL Optimized  Numerator=imag(Taps)  Sharing=off  SharingFactor=2  SimulateUsing=Code generation  roundingMode=Floor  overflowMode=off  CoefficientsDataTypeStr=Inherit: Same word length as input  CoefficientsMin=[]  CoefficientsMax=[]  OutputDataTypeStr=fixdt(1,16,0)  OutputMin=[]  OutputMax=[]  ValidInPort=on  ReadyPort=off
      settings: SourceProductName=DSP System Toolbox  SourceProductBaseCode=DS
  Logical Operator : Logic  Inputs=4  AllPortsSameDT=off  OutDataTypeStr=boolean
  Real-Imag to Complex : RealImagToComplex
  Subtract : Sum  OutDataTypeStr=int16
  Out1 : Outport
  validOut : Outport  Port=2
  wires:
  Add/1 -> Real-Imag to Complex/1
  Subtract/1 -> Real-Imag to Complex/2
  Real-Imag to Complex/1 -> Out1/1
  Discrete FIR Filter HDL Optimized3/1 -> Subtract/2
  Discrete FIR Filter HDL Optimized2/1 -> Subtract/1
  Complex to Real-Imag/2 -> Discrete FIR Filter HDL Optimized1/1, Discrete FIR Filter HDL Optimized2/1
  Discrete FIR Filter HDL Optimized3/2 -> Logical Operator/4
  Discrete FIR Filter HDL Optimized2/2 -> Logical Operator/3
  Complex to Real-Imag/1 -> Discrete FIR Filter HDL Optimized/1, Discrete FIR Filter HDL Optimized3/1
  In1/1 -> Complex to Real-Imag/1
  validIn/1 -> Discrete FIR Filter HDL Optimized/2, Discrete FIR Filter HDL Optimized1/2, Discrete FIR Filter HDL Optimized2/2, Discrete FIR Filter HDL Optimized3/2
  Discrete FIR Filter HDL Optimized1/1 -> Add/2
  Discrete FIR Filter HDL Optimized1/2 -> Logical Operator/2
  Discrete FIR Filter HDL Optimized/2 -> Logical Operator/1
  Logical Operator/1 -> validOut/1
  Discrete FIR Filter HDL Optimized/1 -> Add/1

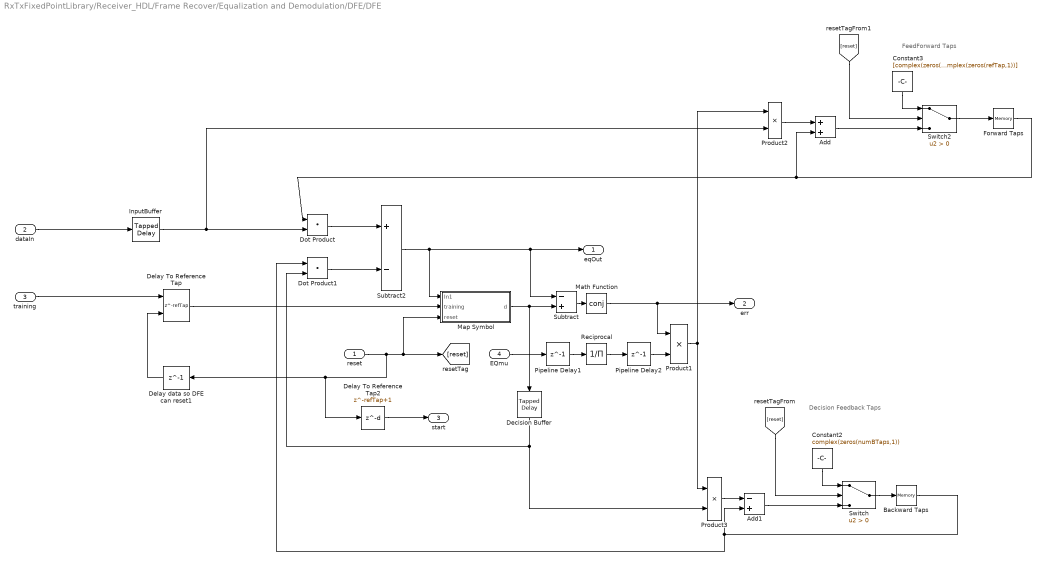
== system RxTxFixedPointLibrary/Receiver_HDL/Frame Recover/Equalization and Demodulation/DFE/DFE ==
  note: Decision Feedback Taps
  note: FeedForward Taps
  reset : Inport
  dataIn : Inport  Port=2  OutDataTypeStr=fixdt(1,16,14)
  training : Inport  Port=3  OutDataTypeStr=fixdt(1,16,15)
  EQmu : Inport  Port=4
  Add : Sum  OutDataTypeStr=fixdt(1,16,14)
  Add1 : Sum  Inputs=-+  OutDataTypeStr=fixdt(1,16,19)
  Backward Taps : Memory  InitialCondition=complex(zeros(numBTaps,1))  InheritSampleTime=on
  Constant2 : Constant  Value=complex(zeros(numBTaps,1))  OutDataTypeStr=fixdt(1,16,4)  SampleTime=-1
  Constant3 : Constant  Value=[complex(zeros(numFTaps-1-refTap,1));1;complex(zeros(refTap,1))]  OutDataTypeStr=fixdt(1,16,4)  SampleTime=-1
  Decision Buffer : simulink/Discrete/Tapped Delay  vinit=0.0  samptime=-1  NumDelays=numBTaps  DelayOrder=Oldest  includeCurrent=off
  Delay To Reference Tap : Delay  DelayLength=refTap  ExternalReset=Level
      settings: InputPortMap=u0,r5
  Delay To Reference Tap2 : Delay  DelayLength=refTap+1
  Delay data so DFE can reset1 : Delay  DelayLength=1
  Dot Product : DotProduct  OutDataTypeStr=fixdt(1,16,14)  SaturateOnIntegerOverflow=on  InputSameDT=on
  Dot Product1 : DotProduct  OutDataTypeStr=fixdt(1,16,18)  SaturateOnIntegerOverflow=on  InputSameDT=on
  Forward Taps : Memory  InitialCondition=[complex(zeros(numFTaps-1-refTap,1));1;complex(zeros(refTap,1))]  InheritSampleTime=on
  InputBuffer : simulink/Discrete/Tapped Delay  vinit=0.0  samptime=-1  NumDelays=numFTaps  DelayOrder=Oldest  includeCurrent=off
  Map Symbol : Subsystem
  Math Function : Math  Operator=conj  RndMeth=Zero  SaturateOnIntegerOverflow=on
  Pipeline Delay1 : Delay  DelayLength=1
  Pipeline Delay2 : Delay  DelayLength=1
  Product1 : Product  OutDataTypeStr=fixdt(1,16,22)
  Product2 : Product  OutDataTypeStr=fixdt(1,16,22)
  Product3 : Product  OutDataTypeStr=fixdt(1,16,21)
  Reciprocal : Product  Inputs=/  OutDataTypeStr=fixdt(0,16,22)  SaturateOnIntegerOverflow=on  RndMeth=Zero
  Subtract : Sum  Inputs=-+  OutDataTypeStr=fixdt(1,16,15)
  Subtract2 : Sum  Inputs=+-  OutDataTypeStr=fixdt(1,16,14)
  Switch : Switch  Criteria=u2 > Threshold  OutDataTypeStr=fixdt(1,16,15)
  Switch2 : Switch  Criteria=u2 > Threshold  OutDataTypeStr=fixdt(1,16,14)
  eqOut : Outport
  err : Outport  Port=2
  start : Outport  Port=3
  wires:
  Math Function/1 -> Product1/1, err/1
  Product1/1 -> Product3/1, Product2/1
  EQmu/1 -> Pipeline Delay1/1
  Pipeline Delay2/1 -> Product1/2
  Pipeline Delay1/1 -> Reciprocal/1
  Reciprocal/1 -> Pipeline Delay2/1
  Delay To Reference Tap2/1 -> start/1
  Delay data so DFE can reset1/1 -> Delay To Reference Tap/2
  Delay To Reference Tap/1 -> Map Symbol/2(training)
  training/1 -> Delay To Reference Tap/1
  dataIn/1 -> InputBuffer/1
  Product3/1 -> Add1/1
  Product2/1 -> Add/1
  [reset] -> Switch2/2
  Constant3/1 -> Switch2/1
  Add/1 -> Switch2/3
  Switch2/1 -> Forward Taps/1
  [reset] -> Switch/2
  Constant2/1 -> Switch/1
  Switch/1 -> Backward Taps/1
  Add1/1 -> Switch/3
  Decision Buffer/1 -> Dot Product1/2, Product3/2
  Backward Taps/1 -> Add1/2, Dot Product1/1
  reset/1 -> Map Symbol/3(reset), [reset], Delay data so DFE can reset1/1, Delay To Reference Tap2/1
  Map Symbol/1(d) -> Decision Buffer/1, Subtract/2
  Forward Taps/1 -> Add/2, Dot Product/1
  Subtract/1 -> Math Function/1
  Subtract2/1 -> eqOut/1, Subtract/1, Map Symbol/1(In1)
  Dot Product1/1 -> Subtract2/2
  Dot Product/1 -> Subtract2/1
  InputBuffer/1 -> Dot Product/2, Product2/2

== system RxTxFixedPointLibrary/Receiver_HDL/Frame Recover/Equalization and Demodulation/DFE/Packeted To Unpacked ==
  In1 : Inport
  Extract Bits : simulink/Logic and Bit Operations/Extract Bits  bitsToExtract=Range of bits  numBits=8  bitIdxRange=[1]  outScalingMode=Treat bit field as an integer
      settings: SourceProductName=Simulink
  Extract Bits1 : simulink/Logic and Bit Operations/Extract Bits  bitsToExtract=Range of bits  numBits=8  bitIdxRange=[0]  outScalingMode=Treat bit field as an integer
      settings: SourceProductName=Simulink
  Vector Concatenate : Concatenate
  Out1 : Outport
  wires:
  Vector Concatenate/1 -> Out1/1
  Extract Bits1/1 -> Vector Concatenate/2
  Extract Bits/1 -> Vector Concatenate/1
  In1/1 -> Extract Bits/1, Extract Bits1/1

== system RxTxFixedPointLibrary/Receiver_HDL/Frame Recover/Gardner Timing Recovery/Gardner TED Blocks/Imag Error ==
  data : Inport
  strobe sum : Inport  Port=2
  Delay : Delay  DelayLength=1
  Product1 : Product
  Sub : Sum  Inputs=+-
  TED Buffer Update1 : Subsystem
  Out1 : Outport
  wires:
  TED Buffer Update1/1(Middle Indx) -> Product1/1
  Delay/1 -> TED Buffer Update1/1(new data)
  TED Buffer Update1/2(oldest) -> Sub/1
  strobe sum/1 -> TED Buffer Update1/2(strobe sum)
  data/1 -> Delay/1, Sub/2
  Sub/1 -> Product1/2
  Product1/1 -> Out1/1

== system RxTxFixedPointLibrary/Receiver_HDL/Frame Recover/Gardner Timing Recovery/Gardner TED Blocks/Real Error ==
  data : Inport
  strobe sum : Inport  Port=2
  Delay : Delay  DelayLength=1
  Product1 : Product  OutDataTypeStr=fixdt(1,16,12)
  Sub : Sum  Inputs=+-
  TED Buffer Update1 : Subsystem
  Out1 : Outport
  wires:
  TED Buffer Update1/1(Middle Indx) -> Product1/1
  Delay/1 -> TED Buffer Update1/1(new data)
  TED Buffer Update1/2(oldest) -> Sub/1
  strobe sum/1 -> TED Buffer Update1/2(strobe sum)
  data/1 -> Delay/1, Sub/2
  Sub/1 -> Product1/2
  Product1/1 -> Out1/1

== system RxTxFixedPointLibrary/Receiver_HDL/Frame Recover/Gardner Timing Recovery/InterpControl_Blocks1/Calculate New mu ==
  note: Good at fixd(0,16,12)
  W : Inport
  NCOCounter : Inport  Port=2
  Math Reciprocal : Math  Operator=reciprocal  OutDataTypeStr=fixdt(1,16,12)  RndMeth=Zero  SaturateOnIntegerOverflow=on
  Product : Product  OutDataTypeStr=fixdt(0,15,14)
  mu : Outport
  wires:
  W/1 -> Math Reciprocal/1
  NCOCounter/1 -> Product/2
  Math Reciprocal/1 -> Product/1
  Product/1 -> mu/1

== system RxTxFixedPointLibrary/Receiver_HDL/Frame Recover/Gardner Timing Recovery/InterpControl_Blocks1/Mod 1 ==
  In1 : Inport
  Add : Sum
  Compare To Constant : simulink/Logic and Bit Operations/Compare To Constant  relop=<  const=1  OutDataTypeStr=boolean
  Compare To Constant1 : simulink/Logic and Bit Operations/Compare To Constant  relop=>=  const=0  OutDataTypeStr=boolean
  Constant : Constant  OutDataTypeStr=fixdt(0,1,0)  SampleTime=-1
  Constant1 : Constant  OutDataTypeStr=fixdt(0,1,0)  SampleTime=-1
  Logical Operator : Logic  AllPortsSameDT=off  OutDataTypeStr=boolean
  Subtract : Sum  Inputs=+-
  Switch : Switch  Criteria=u2 > Threshold
  Switch1 : Switch
  Out1 : Outport
  wires:
  Logical Operator/1 -> Switch/2
  Compare To Constant/1 -> Logical Operator/2
  Compare To Constant1/1 -> Logical Operator/1
  In1/1 -> Subtract/1, Add/1, Switch/1, Compare To Constant/1, Compare To Constant1/1, Switch1/2
  Add/1 -> Switch1/3
  Subtract/1 -> Switch1/1
  Switch1/1 -> Switch/3
  Constant1/1 -> Add/2
  Constant/1 -> Subtract/2
  Switch/1 -> Out1/1

== system RxTxFixedPointLibrary/Receiver_HDL/Frame Recover/Equalization and Demodulation/DFE/DFE/Map Symbol ==
  In1 : Inport  OutDataTypeStr=fixdt(1,16,14)
  training : Inport  Port=2  OutDataTypeStr=fixdt(1,16,15)
  reset : Inport  Port=3
  Decision Directed : Subsystem
  Delay : Delay  DelayLength=1
  HDL Counter : hdlsllib/Sources/HDL Counter  CountType=Count limited  CountInit=0  CountStep=1  CountMax=2^18  CountFromType=Initial value  CountFrom=0  CountResetPort=on  CountLoadPort=off  CountEnbPort=off  CountDirPort=off  CountDataType=Unsigned  CountWordLen=32  CountFracLen=0  CountSampTime=1
      settings: SourceProductBaseCode=HD
  Switch : Switch  Criteria=u2 > Threshold  Threshold=numTrainingSamples  OutDataTypeStr=fixdt(1,16,15)
  d : Outport
  wires:
  Delay/1 -> Switch/3
  training/1 -> Delay/1
  Decision Directed/1(decision) -> Switch/1
  HDL Counter/1 -> Switch/2
  reset/1 -> HDL Counter/1
  Switch/1 -> d/1
  In1/1 -> Decision Directed/1(eqOut)

== system RxTxFixedPointLibrary/Receiver_HDL/Frame Recover/Gardner Timing Recovery/Gardner TED Blocks/Imag Error/TED Buffer Update1 ==
  new data : Inport
  strobe sum : Inport  Port=2
  Delay{,1..3} (4 alike) : Delay  DelayLength=1
  Multiport Switch{,1..3} (4 alike) : MultiPortSwitch  DataPortOrder=Zero-based contiguous  DataPortIndices={0,1,[2,3]}  zeroidx=on
  Zero bit : Constant  Value=0  OutDataTypeStr=fixdt(1,16,13)  SampleTime=1/RadioSampleRate
  Middle Indx : Outport
  oldest : Outport  Port=2
  wires:
  Multiport Switch/1 -> oldest/1, Delay/1
  Multiport Switch3/1 -> Delay3/1
  Multiport Switch2/1 -> Delay2/1, Middle Indx/1
  Multiport Switch1/1 -> Delay1/1
  Delay3/1 -> Multiport Switch3/2, Multiport Switch2/3, Multiport Switch1/4
  Zero bit/1 -> Multiport Switch2/4
  new data/1 -> Multiport Switch3/3, Multiport Switch3/4
  Delay2/1 -> Multiport Switch2/2, Multiport Switch1/3, Multiport Switch/4
  Delay1/1 -> Multiport Switch1/2, Multiport Switch/3
  Delay/1 -> Multiport Switch/2
  strobe sum/1 -> Multiport Switch/1, Multiport Switch1/1, Multiport Switch2/1, Multiport Switch3/1

== system RxTxFixedPointLibrary/Receiver_HDL/Frame Recover/Gardner Timing Recovery/Gardner TED Blocks/Real Error/TED Buffer Update1 ==
  new data : Inport
  strobe sum : Inport  Port=2
  Delay{,1..3} (4 alike) : Delay  DelayLength=1
  Multiport Switch{,1..3} (4 alike) : MultiPortSwitch  DataPortOrder=Zero-based contiguous  DataPortIndices={0,1,[2,3]}  zeroidx=on
  Zero bit : Constant  Value=0  OutDataTypeStr=fixdt(1,16,13)  SampleTime=1/RadioSampleRate
  Middle Indx : Outport
  oldest : Outport  Port=2
  wires:
  Multiport Switch/1 -> oldest/1, Delay/1
  Multiport Switch3/1 -> Delay3/1
  Multiport Switch2/1 -> Delay2/1, Middle Indx/1
  Multiport Switch1/1 -> Delay1/1
  Delay3/1 -> Multiport Switch3/2, Multiport Switch2/3, Multiport Switch1/4
  Zero bit/1 -> Multiport Switch2/4
  new data/1 -> Multiport Switch3/3, Multiport Switch3/4
  Delay2/1 -> Multiport Switch2/2, Multiport Switch1/3, Multiport Switch/4
  Delay1/1 -> Multiport Switch1/2, Multiport Switch/3
  Delay/1 -> Multiport Switch/2
  strobe sum/1 -> Multiport Switch/1, Multiport Switch1/1, Multiport Switch2/1, Multiport Switch3/1

== system RxTxFixedPointLibrary/Receiver_HDL/Frame Recover/Equalization and Demodulation/DFE/DFE/Map Symbol/Decision Directed ==
  eqOut : Inport  OutDataTypeStr=fixdt(1,16,14)
  Compare To Zero : simulink/Logic and Bit Operations/Compare To Zero  relop=>=  OutDataTypeStr=boolean
  Compare To Zero1 : simulink/Logic and Bit Operations/Compare To Zero  relop=>=  OutDataTypeStr=boolean
  Complex to Real-Imag : ComplexToRealImag
  QPSK Decisions : LookupNDDirect  Table=[-0.7071 - 0.7071i, -0.7071 + 0.7071i; 0.7071 - 0.7071i, 0.7071 + 0.7071i]  DiagnosticForOutOfRangeInput=Error  TableDataTypeStr=fixdt(1,16,15)
  decision : Outport
  wires:
  QPSK Decisions/1 -> decision/1
  Compare To Zero1/1 -> QPSK Decisions/2
  Compare To Zero/1 -> QPSK Decisions/1
  Complex to Real-Imag/2 -> Compare To Zero1/1
  Complex to Real-Imag/1 -> Compare To Zero/1
  eqOut/1 -> Complex to Real-Imag/1

== matlab function RxTxFixedPointLibrary/Receiver_HDL/Frame Recover/Frequency Recovery/Lock Detector/MATLAB Function ==
  data: u input; y output
function y = abs(u)

y = fi(u,0,16,10);
